simulink model "steps"  (Simulink 6.0)
settings: Solver=ode45  SolverMode=SingleTasking  StartTime=0.0  StopTime=10000  MaxStep=5  RelTol=1e-3  AbsTol=1e-6
settings Model: Creator=The MathWorks Inc.  LastModifiedBy=batserve  ExtModeTrigMode=oneshot  ExtModeAutoUpdateStatusClock=off
settings DataIOCC: ExternalInput=[]  InitialState=[]  LimitDataPoints=off  SaveOutput=off  SaveTime=off
settings OptimizationCC: BooleanDataType=off
settings DebuggingCC: CheckExecutionContextPreStartOutputMsg=on  CheckExecutionContextRuntimeOutputMsg=on  SolverPrmCheckMsg=none
settings HardwareCC: TargetUnknown=on

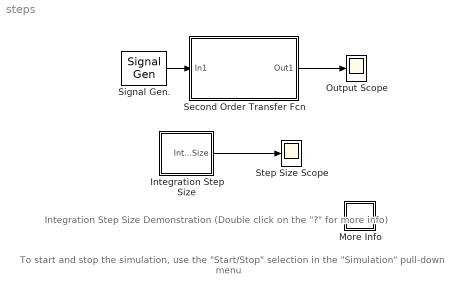
== system steps ==
  note: To start and stop the simulation, use the "Start/Stop"
      | selection in the "Simulation" pull-down menu
  note: Integration Step Size Demonstration
      | (Double click on the "?" for more info)
  Integration Step Size : Subsystem  PropExecContextAcrossSSBoundary=on
      mask Display: plot(0,0,100,100,[90,69,69,49,49,27,27,10],[74,74,60,60,40,40,80,80],[27,27],[10,30],[49,49],[10,30],[27,49,49,27],[19,19,21,21])
  More Info : Subsystem  PropExecContextAcrossSSBoundary=on
      mask Display: disp('?')
  Output Scope : Scope
      settings: TickLabels=on  TimeRange=40  YMin=-0.75  YMax=0.75  DataFormat=Array
  Second Order Transfer Fcn : Subsystem  PropExecContextAcrossSSBoundary=on  mask(Mass-Spring-Damper System){@1=2, @2=0.5}
      mask prompts: @1 "Natural Frequency (rad/sec)"; @2 "Damping"
      mask help: Mass-Spring-Damper System
      mask init:
      | w=@1;zeta=@2;
      mask Help: This block implements the second order transfer function G(s)=num(s)/den(2) where num(s)=w^2 and den(s)=[1 2*zeta*w w^2].
      mask Display: disp('Mass-Spring\nDamper System')
  Signal Gen. : SignalGenerator  WaveForm=square  Frequency=0.500000
  Step Size Scope : Scope
      settings: TickLabels=on  TimeRange=40  YMin=-2.77556e-17  YMax=0.35  DataFormat=Array
  wires:
  Signal Gen./1 -> Second Order Transfer Fcn/1(In1)
  Second Order Transfer Fcn/1(Out1) -> Output Scope/1
  Integration Step Size/1(Integration Step Size) -> Step Size Scope/1

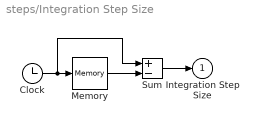
== system steps/Integration Step Size ==
  Clock : Clock
      settings: Decimation=10
  Memory : Memory
  Sum : Sum  Inputs=+-  SaturateOnIntegerOverflow=on  InputSameDT=on
  Integration Step Size : Outport  InitialOutput=0
  wires:
  Memory/1 -> Sum/2
  Clock/1 -> Memory/1, Sum/1
  Sum/1 -> Integration Step Size/1

== system steps/More Info ==
  note: Try changing the natural frequency and damping
      | of this system. You might also try changing the
      | integration algorithm (in the "Parameters..." dialog
      | under the "Simulation" pull-down menu) to see
      | the effect on integration step size.
  note: This model simulates a second order
      | mass-spring-damper system. The lower of
      | the two scope blocks shows the integration
      | step size of the current integration algorithm.

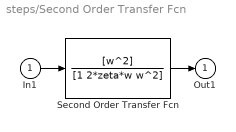
== system steps/Second Order Transfer Fcn ==
  In1 : Inport  Port=1  LatchInput=off
  Second Order Transfer Fcn : TransferFcn  Numerator=[w^2]  Denominator=[1 2*zeta*w w^2]
  Out1 : Outport  InitialOutput=0
  wires:
  Second Order Transfer Fcn/1 -> Out1/1
  In1/1 -> Second Order Transfer Fcn/1
